simulink model "Lab14ContDisc_2018a1"  (R2018a)
settings: Solver=ode45  StartTime=0.0  StopTime=100  RelTol=1e-3  EnableMultiTasking=on
libraries: cstblocks x2
settings Model: Creator=morai  LastModifiedBy=Adm
settings DataIOCC: LimitDataPoints=on
settings OptimizationCC: LifeSpan=inf
settings DebuggingCC: AllowSymbolicDim=off  SFUnexpectedBacktrackingDiag=warning  SFNoUnconditionalDefaultTransitionDiag=warning  SFExecutionAtInitializationDiag=none
settings ModelReferenceCC: PropagateSignalLabelsOutOfModel=off
settings CodeAppCC: StateflowObjectComments=on
settings GRTTargetCC: TargetLangStandard=C89/C90 (ANSI)
settings ConfigComp: CovMetricSettings=dw  CovSaveCumulativeToWorkspaceVar=on  CovSaveSingleToWorkspaceVar=on  CovExternalEMLEnable=off

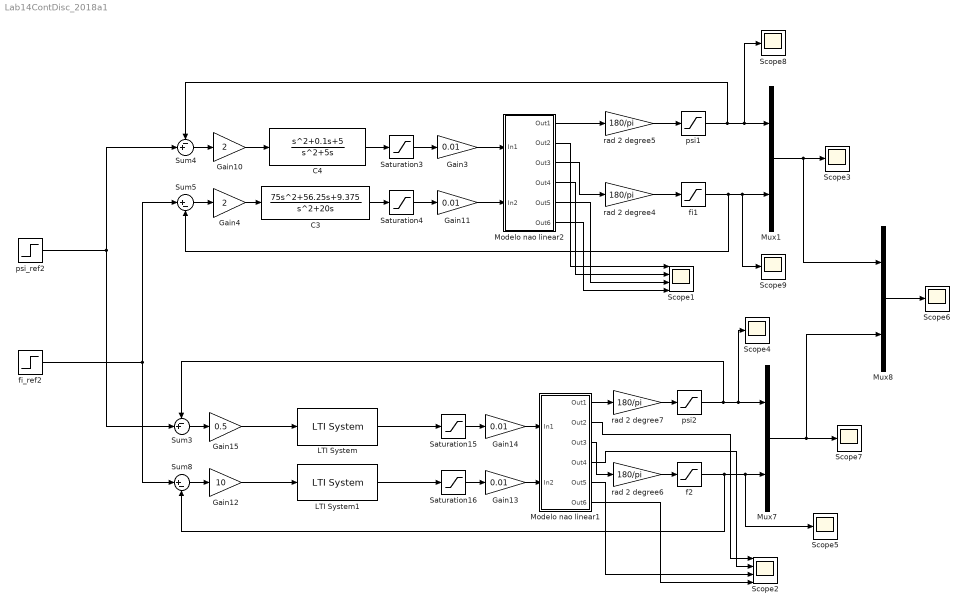
== system Lab14ContDisc_2018a1 ==
  C3 : TransferFcn  Numerator=[75 56.25 9.375]  Denominator=[1 20 0]
  C4 : TransferFcn  Numerator=[1 0.1 5]  Denominator=[1 5 0]
  Gain10 : Gain  Gain=2
  Gain{3,11,13..14} (4 alike) : Gain  Gain=0.01
  Gain12 : Gain  Gain=10
  Gain15 : Gain  Gain=0.5
  Gain4 : Gain  Gain=2
  LTI System : cstblocks/LTI System  sys=C1z  IC=[]
  LTI System1 : cstblocks/LTI System  sys=C2z  IC=[]
  Modelo nao linear1 : Subsystem
  Modelo nao linear2 : Subsystem
  Mux1 : Mux  Inputs=2
  Mux7 : Mux  Inputs=2
  Mux8 : Mux  Inputs=2
  Saturation{3..4,15..16} (4 alike) : Saturate  UpperLimit=255  LowerLimit=-255
  Scope1 : Scope  NumInputPorts=4
  Scope2 : Scope  NumInputPorts=4
  Scope{3..9} (7 alike) : Scope
  Sum3 : Sum  Inputs=-+|
  Sum4 : Sum  Inputs=-+|
  Sum5 : Sum  Inputs=|+-
  Sum8 : Sum  Inputs=|+-
  f2 : Saturate  UpperLimit=180  LowerLimit=-180
  fi1 : Saturate  UpperLimit=180  LowerLimit=-180
  fi_ref2 : Step  Time=70  Before=160  After=50  SampleTime=0
  psi1 : Saturate  UpperLimit=80  LowerLimit=-80
  psi2 : Saturate  UpperLimit=80  LowerLimit=-80
  psi_ref2 : Step  Time=40  Before=-32  After=0  SampleTime=0
  rad 2 degree{4..7} (4 alike) : Gain  Gain=180/pi
  wires:
  Gain14/1 -> Modelo nao linear1/1(In1)
  psi2/1 -> Scope4/1, Mux7/1, Sum3/1
  rad 2 degree6/1 -> f2/1
  Saturation16/1 -> Gain13/1
  C3/1 -> Saturation4/1
  Modelo nao linear1/1(Out1) -> rad 2 degree7/1
  Gain10/1 -> C4/1
  Saturation15/1 -> Gain14/1
  Gain4/1 -> C3/1
  Sum4/1 -> Gain10/1
  Gain13/1 -> Modelo nao linear1/2(In2)
  Mux8/1 -> Scope6/1
  f2/1 -> Sum8/2, Scope5/1, Mux7/2
  fi1/1 -> Sum5/2, Scope9/1, Mux1/2
  Saturation4/1 -> Gain11/1
  Saturation3/1 -> Gain3/1
  Gain15/1 -> LTI System/1
  Sum3/1 -> Gain15/1
  LTI System/1 -> Saturation15/1
  rad 2 degree7/1 -> psi2/1
  C4/1 -> Saturation3/1
  Mux1/1 -> Scope3/1, Mux8/1
  Sum8/1 -> Gain12/1
  Sum5/1 -> Gain4/1
  rad 2 degree4/1 -> fi1/1
  Gain11/1 -> Modelo nao linear2/2(In2)
  LTI System1/1 -> Saturation16/1
  psi1/1 -> Scope8/1, Mux1/1, Sum4/1
  Modelo nao linear1/3(Out3) -> rad 2 degree6/1
  Gain3/1 -> Modelo nao linear2/1(In1)
  Mux7/1 -> Mux8/2, Scope7/1
  rad 2 degree5/1 -> psi1/1
  Gain12/1 -> LTI System1/1
  psi_ref2/1 -> Sum3/2, Sum4/2
  fi_ref2/1 -> Sum5/1, Sum8/1
  Modelo nao linear2/3(Out3) -> rad 2 degree4/1
  Modelo nao linear2/1(Out1) -> rad 2 degree5/1
  Modelo nao linear1/6(Out6) -> Scope2/4
  Modelo nao linear1/5(Out5) -> Scope2/3
  Modelo nao linear1/4(Out4) -> Scope2/2
  Modelo nao linear1/2(Out2) -> Scope2/1
  Modelo nao linear2/2(Out2) -> Scope1/1
  Modelo nao linear2/4(Out4) -> Scope1/2
  Modelo nao linear2/5(Out5) -> Scope1/3
  Modelo nao linear2/6(Out6) -> Scope1/4

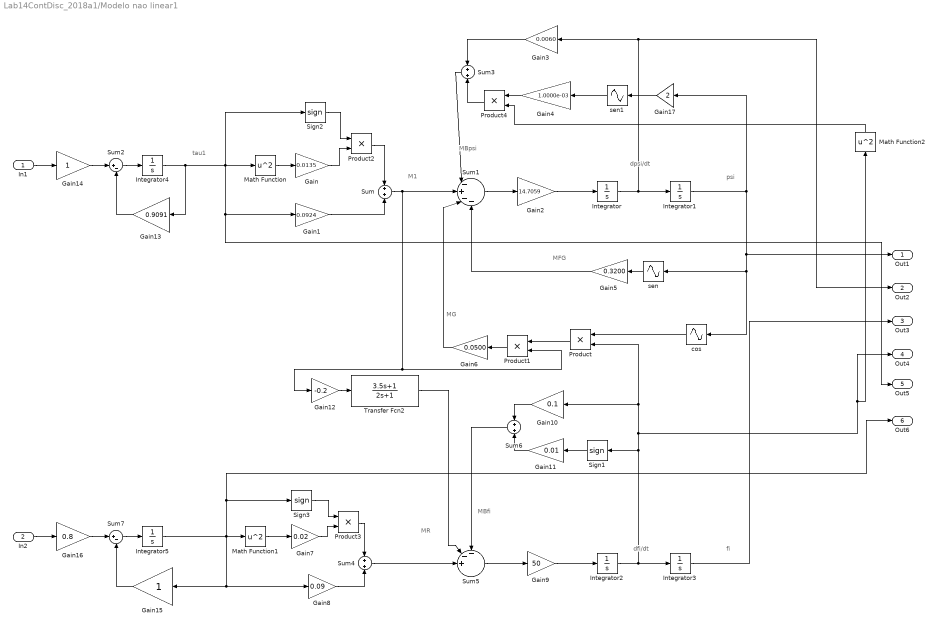
== system Lab14ContDisc_2018a1/Modelo nao linear1 ==
  note: MBfi
  note: MR
  note: psi
  note: MFG
  note: tau1
  note: M1
  note: MG
  note: MBpsi
  note: fi
  note: dfi/dt
  note: dpsi/dt
  In1 : Inport
  In2 : Inport  Port=2
  Gain : Gain  Gain=0.0135
  Gain1 : Gain  Gain=0.0924
  Gain10 : Gain  Gain=0.1
  Gain11 : Gain  Gain=0.01
  Gain12 : Gain  Gain=-0.2
  Gain13 : Gain  Gain=0.9091
  Gain14 : Gain
  Gain15 : Gain
  Gain16 : Gain  Gain=0.8
  Gain17 : Gain  Gain=2
  Gain2 : Gain  Gain=14.7059
  Gain3 : Gain  Gain=0.0060
  Gain4 : Gain  Gain=1.0000e-03
  Gain5 : Gain  Gain=0.3200
  Gain6 : Gain  Gain=0.0500
  Gain7 : Gain  Gain=0.02
  Gain8 : Gain  Gain=0.09
  Gain9 : Gain  Gain=50
  Integrator{,1..5} (6 alike) : Integrator
  Math Function : Math  Operator=square  SaturateOnIntegerOverflow=on
  Math Function1 : Math  Operator=square  SaturateOnIntegerOverflow=on
  Math Function2 : Math  Operator=square  SaturateOnIntegerOverflow=on
  Product{,1..4} (5 alike) : Product
  Sign1 : Signum  ZeroCross=off
  Sign2 : Signum  ZeroCross=off
  Sign3 : Signum  ZeroCross=off
  Sum{,3..4,6} (4 alike) : Sum
  Sum1 : Sum  Inputs=|-+--
  Sum2 : Sum  Inputs=|+-
  Sum5 : Sum  Inputs=--+||
  Sum7 : Sum  Inputs=|+-
  Transfer Fcn2 : TransferFcn  Numerator=[3.5 1]  Denominator=[2 1]
  cos : Sin  TimeSource=Use external signal  Phase=pi/2  SampleTime=0
  sen : Sin  TimeSource=Use external signal  SampleTime=0
  sen1 : Sin  TimeSource=Use external signal  SampleTime=0
  Out1 : Outport
  Out2 : Outport  Port=2
  Out3 : Outport  Port=3
  Out4 : Outport  Port=4
  Out5 : Outport  Port=5
  Out6 : Outport  Port=6
  wires:
  Gain14/1 -> Sum2/1
  Integrator5/1 -> Math Function1/1, Sign3/1, Out6/1, Gain8/1, Gain15/1
  Sum2/1 -> Integrator4/1
  Gain15/1 -> Sum7/2
  Gain13/1 -> Sum2/2
  In1/1 -> Gain14/1
  Gain16/1 -> Sum7/1
  Sum7/1 -> Integrator5/1
  Integrator4/1 -> Gain13/1, Sign2/1, Math Function/1, Out5/1, Gain1/1
  Math Function/1 -> Gain/1
  Gain1/1 -> Sum/2
  Sum1/1 -> Gain2/1
  Gain2/1 -> Integrator/1
  Gain3/1 -> Sum3/1
  Sum3/1 -> Sum1/1
  Sum/1 -> Product1/2, Gain12/1, Sum1/2
  Integrator1/1 -> cos/1, sen/1, Out1/1, Gain17/1
  sen/1 -> Gain5/1
  Gain5/1 -> Sum1/4
  cos/1 -> Product/1
  Integrator2/1 -> Product/2, Gain10/1, Out4/1, Math Function2/1, Sign1/1, Integrator3/1
  Product1/1 -> Gain6/1
  Gain6/1 -> Sum1/3
  Product/1 -> Product1/1
  Math Function1/1 -> Gain7/1
  Gain8/1 -> Sum4/2
  Sum5/1 -> Gain9/1
  Gain9/1 -> Integrator2/1
  Sign1/1 -> Gain11/1
  Gain10/1 -> Sum6/1
  Gain11/1 -> Sum6/2
  In2/1 -> Gain16/1
  Integrator3/1 -> Out3/1
  Sum4/1 -> Sum5/3
  Sum6/1 -> Sum5/1
  Transfer Fcn2/1 -> Sum5/2
  Gain12/1 -> Transfer Fcn2/1
  Sign2/1 -> Product2/1
  Gain/1 -> Product2/2
  Product2/1 -> Sum/1
  Gain7/1 -> Product3/2
  Sign3/1 -> Product3/1
  Product3/1 -> Sum4/1
  sen1/1 -> Gain4/1
  Gain17/1 -> sen1/1
  Integrator/1 -> Out2/1, Gain3/1, Integrator1/1
  Gain4/1 -> Product4/1
  Product4/1 -> Sum3/2
  Math Function2/1 -> Product4/2

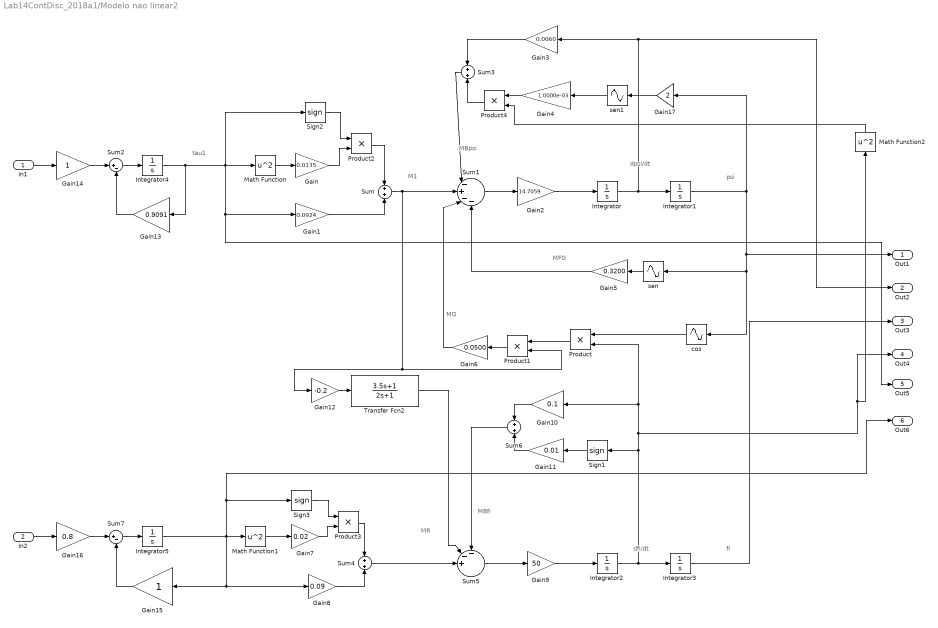
== system Lab14ContDisc_2018a1/Modelo nao linear2 ==
  note: MBfi
  note: MR
  note: psi
  note: MFG
  note: tau1
  note: M1
  note: MG
  note: MBpsi
  note: fi
  note: dfi/dt
  note: dpsi/dt
  In1 : Inport
  In2 : Inport  Port=2
  Gain : Gain  Gain=0.0135
  Gain1 : Gain  Gain=0.0924
  Gain10 : Gain  Gain=0.1
  Gain11 : Gain  Gain=0.01
  Gain12 : Gain  Gain=-0.2
  Gain13 : Gain  Gain=0.9091
  Gain14 : Gain
  Gain15 : Gain
  Gain16 : Gain  Gain=0.8
  Gain17 : Gain  Gain=2
  Gain2 : Gain  Gain=14.7059
  Gain3 : Gain  Gain=0.0060
  Gain4 : Gain  Gain=1.0000e-03
  Gain5 : Gain  Gain=0.3200
  Gain6 : Gain  Gain=0.0500
  Gain7 : Gain  Gain=0.02
  Gain8 : Gain  Gain=0.09
  Gain9 : Gain  Gain=50
  Integrator{,1..5} (6 alike) : Integrator
  Math Function : Math  Operator=square  SaturateOnIntegerOverflow=on
  Math Function1 : Math  Operator=square  SaturateOnIntegerOverflow=on
  Math Function2 : Math  Operator=square  SaturateOnIntegerOverflow=on
  Product{,1..4} (5 alike) : Product
  Sign1 : Signum  ZeroCross=off
  Sign2 : Signum  ZeroCross=off
  Sign3 : Signum  ZeroCross=off
  Sum{,3..4,6} (4 alike) : Sum
  Sum1 : Sum  Inputs=|-+--
  Sum2 : Sum  Inputs=|+-
  Sum5 : Sum  Inputs=--+||
  Sum7 : Sum  Inputs=|+-
  Transfer Fcn2 : TransferFcn  Numerator=[3.5 1]  Denominator=[2 1]
  cos : Sin  TimeSource=Use external signal  Phase=pi/2  SampleTime=0
  sen : Sin  TimeSource=Use external signal  SampleTime=0
  sen1 : Sin  TimeSource=Use external signal  SampleTime=0
  Out1 : Outport
  Out2 : Outport  Port=2
  Out3 : Outport  Port=3
  Out4 : Outport  Port=4
  Out5 : Outport  Port=5
  Out6 : Outport  Port=6
  wires:
  Gain14/1 -> Sum2/1
  Integrator5/1 -> Math Function1/1, Sign3/1, Out6/1, Gain8/1, Gain15/1
  Sum2/1 -> Integrator4/1
  Gain15/1 -> Sum7/2
  Gain13/1 -> Sum2/2
  In1/1 -> Gain14/1
  Gain16/1 -> Sum7/1
  Sum7/1 -> Integrator5/1
  Integrator4/1 -> Gain13/1, Sign2/1, Math Function/1, Out5/1, Gain1/1
  Math Function/1 -> Gain/1
  Gain1/1 -> Sum/2
  Sum1/1 -> Gain2/1
  Gain2/1 -> Integrator/1
  Gain3/1 -> Sum3/1
  Sum3/1 -> Sum1/1
  Sum/1 -> Product1/2, Gain12/1, Sum1/2
  Integrator1/1 -> cos/1, sen/1, Out1/1, Gain17/1
  sen/1 -> Gain5/1
  Gain5/1 -> Sum1/4
  cos/1 -> Product/1
  Integrator2/1 -> Product/2, Gain10/1, Out4/1, Math Function2/1, Sign1/1, Integrator3/1
  Product1/1 -> Gain6/1
  Gain6/1 -> Sum1/3
  Product/1 -> Product1/1
  Math Function1/1 -> Gain7/1
  Gain8/1 -> Sum4/2
  Sum5/1 -> Gain9/1
  Gain9/1 -> Integrator2/1
  Sign1/1 -> Gain11/1
  Gain10/1 -> Sum6/1
  Gain11/1 -> Sum6/2
  In2/1 -> Gain16/1
  Integrator3/1 -> Out3/1
  Sum4/1 -> Sum5/3
  Sum6/1 -> Sum5/1
  Transfer Fcn2/1 -> Sum5/2
  Gain12/1 -> Transfer Fcn2/1
  Sign2/1 -> Product2/1
  Gain/1 -> Product2/2
  Product2/1 -> Sum/1
  Gain7/1 -> Product3/2
  Sign3/1 -> Product3/1
  Product3/1 -> Sum4/1
  sen1/1 -> Gain4/1
  Gain17/1 -> sen1/1
  Integrator/1 -> Out2/1, Gain3/1, Integrator1/1
  Gain4/1 -> Product4/1
  Product4/1 -> Sum3/2
  Math Function2/1 -> Product4/2
